simulink model "SWC04_HVPS_DCDCCntrl"  (R2020b)
settings: Solver=FixedStepDiscrete  StartTime=0.0  StopTime=10.0  FixedStep=0.01  RelTol=1e-3
model workspace (MAT data in the model file):
  KSWC07_PDOff_V = Simulink.Parameter
  KSWC07_PDOff_V.Value = 45
  KSWC07_PDOff_V.DataType = 'uint8'
  KSWC07_PDOff_V.Dimensions = [1 1]
  KSWC07_PDOn_V = Simulink.Parameter
  KSWC07_PDOn_V.Value = 15
  KSWC07_PDOn_V.DataType = 'uint8'
  KSWC07_PDOn_V.Dimensions = [1 1]
  NSWC04_B2VSOCEmgncyChgLow_per = Simulink.Parameter
  NSWC04_B2VSOCEmgncyChgLow_per.Value = 30
  NSWC04_B2VSOCEmgncyChgLow_per.DataType = 'uint8'
  NSWC04_B2VSOCEmgncyChgLow_per.Min = 0
  NSWC04_B2VSOCEmgncyChgLow_per.Max = 100
  NSWC04_B2VSOCEmgncyChgLow_per.Dimensions = [1 1]
  NSWC04_KL30EmgncyChgLow_V = Simulink.Parameter
  NSWC04_KL30EmgncyChgLow_V.Value = 95
  NSWC04_KL30EmgncyChgLow_V.DataType = 'uint8'
  NSWC04_KL30EmgncyChgLow_V.Min = 0
  NSWC04_KL30EmgncyChgLow_V.Max = 240
  NSWC04_KL30EmgncyChgLow_V.Dimensions = [1 1]
undefined symbols (not defined in the file): DCDC_14V, HV240V, HV420V, MCUMd_AD, MCUMd_SB, MFbTrq_Off, MRtt_Off, VhSpd_Off, VSUStt_HVOff, VSUStt_HVOn
libraries: simulink x2
settings Model: OrderedModelArguments=off  Creator=Eric  LastModifiedBy=cyw40
settings OptimizationCC: BlockReduction=off  DefaultParameterBehavior=Inlined  UseDivisionForNetSlopeComputation=on  EnhancedBackFolding=on  PassReuseOutputArgsAs=Individual arguments  EfficientFloat2IntCast=on  OptimizeBlockOrder=speed  DifferentSizesBufferReuse=on  OptimizationCustomize=off  EfficientTunableParamExpr=on
settings DebuggingCC: SignalInfNanChecking=error  SignalRangeChecking=error  ReadBeforeWriteMsg=EnableAllAsError  WriteAfterWriteMsg=EnableAllAsError  WriteAfterReadMsg=EnableAllAsError  AlgebraicLoopMsg=error  ArtificialAlgebraicLoopMsg=error  SaveWithDisabledLinksMsg=error  SaveWithParameterizedLinksMsg=error  BlockPriorityViolationMsg=error  SolverPrmCheckMsg=error  InheritedTsInSrcMsg=error  SingleTaskRateTransMsg=error  TasksWithSamePriorityMsg=error  SigSpecEnsureSampleTimeMsg=error  CheckMatrixSingularityMsg=error  IntegerOverflowMsg=error  ParameterUnderflowMsg=error  ParameterPrecisionLossMsg=error  ParameterTunabilityLossMsg=error  UnderSpecifiedDataTypeMsg=error  UnnecessaryDatatypeConvMsg=warning  VectorMatrixConversionMsg=error  SignalLabelMismatchMsg=error  UnconnectedInputMsg=error  UnconnectedOutputMsg=error  UnconnectedLineMsg=error  SFcnCompatibilityMsg=error  UniqueDataStoreMsg=error  BusObjectLabelMismatch=error  RootOutportRequireBusObject=error  AssertControl=DisableAll  ModelReferenceIOMsg=error  ModelReferenceIOMismatchMessage=error  UnknownTsInhSupMsg=error  ModelReferenceDataLoggingMessage=error  StateNameClashWarn=warning  StrictBusMsg=ErrorOnBusTreatedAsVector  NonBusSignalsTreatedAsBus=error  SFInvalidInputDataAccessInChartInitDiag=error  SFTransitionOutsideNaturalParentDiag=error  SFUnreachableExecutionPathDiag=error  SFUndirectedBroadcastEventsDiag=error  SFTransitionActionBeforeConditionDiag=error  SFTemporalDelaySmallerThanSampleTimeDiag=error  SFSelfTransitionDiag=error  SFExecutionAtInitializationDiag=error  SFMachineParentedDataDiag=error  IntegerSaturationMsg=error
settings SFSimCC: CompileTimeRecursionLimit=0  EnableRuntimeRecursion=off  MATLABDynamicMemAlloc=off
settings RTWCC: Description=Embedded Coder  SystemTargetFile=ert.tlc  TemplateMakefile=ert_default_tmf
settings CodeAppCC: ForceParamTrailComments=on  IgnoreCustomStorageClasses=off  OperatorAnnotations=on  SimulinkDataObjDesc=on  SFDataObjDesc=on  MangleLength=4  InsertBlockDesc=on  ReqsInCode=on
settings ERTTargetCC: TargetLangStandard=C99 (ISO)  GenerateSampleERTMain=on  InlinedParameterPlacement=NonHierarchical  ERTCustomFileTemplate=example_file_process.tlc
settings ConfigComp: DVMode=DesignErrorDetection  DVTestSuiteOptimization=Auto  DVDetectDeadLogic=on  DVDetectActiveLogic=on  DVDetectDivisionByZero=off  DVDetectIntegerOverflow=off

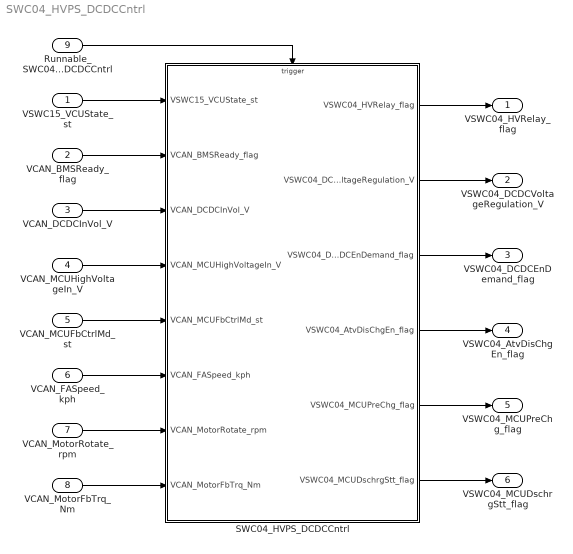
== system SWC04_HVPS_DCDCCntrl ==
  VSWC15_VCUState_st : Inport  OutMin=0  OutMax=13  OutDataTypeStr=uint8  PortDimensions=1
  VCAN_BMSReady_flag : Inport  Port=2  OutMin=0  OutMax=1  OutDataTypeStr=boolean  PortDimensions=1
  VCAN_DCDCInVol_V : Inport  Port=3  OutMin=0  OutMax=500  OutDataTypeStr=uint16  Unit=V  PortDimensions=1
  VCAN_MCUHighVoltageIn_V : Inport  Port=4  OutMin=0  OutMax=500  OutDataTypeStr=uint16  Unit=V  PortDimensions=1
  VCAN_MCUFbCtrlMd_st : Inport  Port=5  OutMin=0  OutMax=4  OutDataTypeStr=uint8  PortDimensions=1
  VCAN_FASpeed_kph : Inport  Port=6  OutMin=0  OutMax=150  OutDataTypeStr=uint8  Unit=km/hr  PortDimensions=1
  VCAN_MotorRotate_rpm : Inport  Port=7  OutMin=0  OutMax=16000  OutDataTypeStr=uint16  Unit=rpm  PortDimensions=1
  VCAN_MotorFbTrq_Nm : Inport  Port=8  OutMin=0  OutMax=225  OutDataTypeStr=uint8  Unit=N*m  PortDimensions=1
  Runnable_SWC04HVPSDCDCCntrl : Inport  Port=9  OutputFunctionCall=on
  SWC04_HVPS_DCDCCntrl : Subsystem
  VSWC04_HVRelay_flag : Outport  OutMin=0  OutMax=1  OutDataTypeStr=boolean  PortDimensions=1
  VSWC04_DCDCVoltageRegulation_V : Outport  Port=2  OutMin=0  OutMax=36  OutDataTypeStr=uint8  Unit=V  PortDimensions=1
  VSWC04_DCDCEnDemand_flag : Outport  Port=3  OutMin=0  OutMax=1  OutDataTypeStr=boolean  PortDimensions=1
  VSWC04_AtvDisChgEn_flag : Outport  Port=4  OutMin=0  OutMax=1  OutDataTypeStr=boolean  PortDimensions=1
  VSWC04_MCUPreChg_flag : Outport  Port=5  OutMin=0  OutMax=1  OutDataTypeStr=boolean  PortDimensions=1
  VSWC04_MCUDschrgStt_flag : Outport  Port=6  OutMin=0  OutMax=1  OutDataTypeStr=boolean  PortDimensions=1
  wires:
  VCAN_BMSReady_flag/1 -> SWC04_HVPS_DCDCCntrl/2(VCAN_BMSReady_flag)
  VCAN_DCDCInVol_V/1 -> SWC04_HVPS_DCDCCntrl/3(VCAN_DCDCInVol_V)
  SWC04_HVPS_DCDCCntrl/2(VSWC04_DCDCVoltageRegulation_V) -> VSWC04_DCDCVoltageRegulation_V/1
  SWC04_HVPS_DCDCCntrl/3(VSWC04_DCDCEnDemand_flag) -> VSWC04_DCDCEnDemand_flag/1
  Runnable_SWC04HVPSDCDCCntrl/1 -> SWC04_HVPS_DCDCCntrl/Trigger
  VSWC15_VCUState_st/1 -> SWC04_HVPS_DCDCCntrl/1(VSWC15_VCUState_st)
  VCAN_MCUHighVoltageIn_V/1 -> SWC04_HVPS_DCDCCntrl/4(VCAN_MCUHighVoltageIn_V)
  SWC04_HVPS_DCDCCntrl/6(VSWC04_MCUDschrgStt_flag) -> VSWC04_MCUDschrgStt_flag/1
  VCAN_MCUFbCtrlMd_st/1 -> SWC04_HVPS_DCDCCntrl/5(VCAN_MCUFbCtrlMd_st)
  SWC04_HVPS_DCDCCntrl/1(VSWC04_HVRelay_flag) -> VSWC04_HVRelay_flag/1
  SWC04_HVPS_DCDCCntrl/5(VSWC04_MCUPreChg_flag) -> VSWC04_MCUPreChg_flag/1
  SWC04_HVPS_DCDCCntrl/4(VSWC04_AtvDisChgEn_flag) -> VSWC04_AtvDisChgEn_flag/1
  VCAN_FASpeed_kph/1 -> SWC04_HVPS_DCDCCntrl/6(VCAN_FASpeed_kph)
  VCAN_MotorRotate_rpm/1 -> SWC04_HVPS_DCDCCntrl/7(VCAN_MotorRotate_rpm)
  VCAN_MotorFbTrq_Nm/1 -> SWC04_HVPS_DCDCCntrl/8(VCAN_MotorFbTrq_Nm)

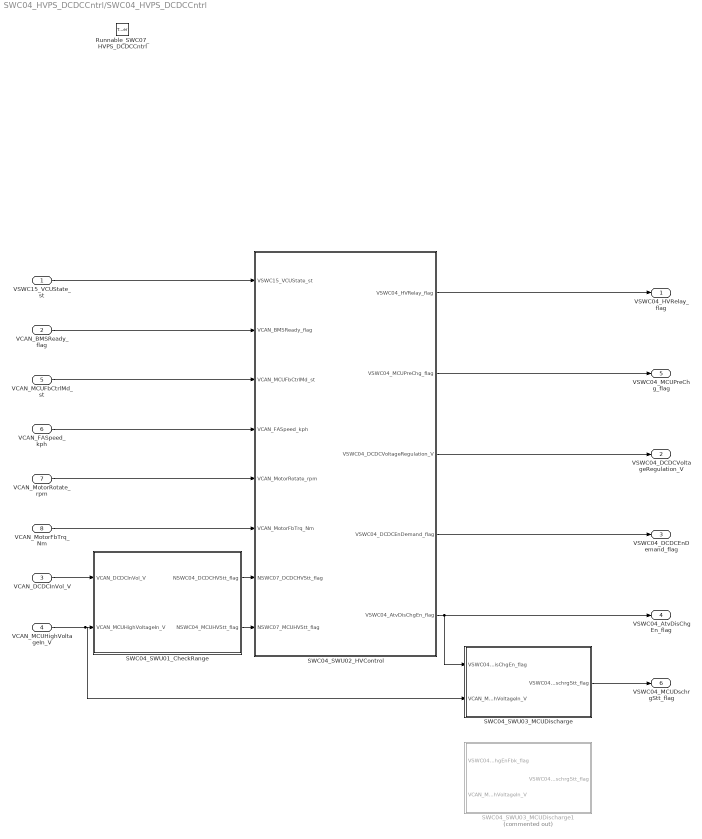
== system SWC04_HVPS_DCDCCntrl/SWC04_HVPS_DCDCCntrl ==
  VSWC15_VCUState_st : Inport
  VCAN_BMSReady_flag : Inport  Port=2
  VCAN_DCDCInVol_V : Inport  Port=3
  VCAN_MCUHighVoltageIn_V : Inport  Port=4
  VCAN_MCUFbCtrlMd_st : Inport  Port=5
  VCAN_FASpeed_kph : Inport  Port=6
  VCAN_MotorRotate_rpm : Inport  Port=7
  VCAN_MotorFbTrq_Nm : Inport  Port=8
  Runnable_SWC07_HVPS_DCDCCntrl : TriggerPort  TriggerType=function-call  VariantControl=Variant
  SWC04_SWU01_CheckRange : Subsystem  TreatAsAtomicUnit=on  RTWFcnName=SWC04_SWU01_CheckRange
      settings: RTWSystemCode=Nonreusable function  RTWFcnNameOpts=User specified
  SWC04_SWU02_HVControl : Subsystem  TreatAsAtomicUnit=on  RTWFcnName=SWC04_SWU02_HVControl
      settings: RTWSystemCode=Nonreusable function  RTWFcnNameOpts=User specified
  SWC04_SWU03_MCUDischarge : Subsystem  TreatAsAtomicUnit=on  RTWFcnName=SWC04_SWU03_MCUDischarge  VariantControl=Choice_1
      settings: RTWSystemCode=Nonreusable function  RTWFcnNameOpts=User specified
  SWC04_SWU03_MCUDischarge1 : Subsystem  Commented=on  VariantControl=Choice_2
  VSWC04_HVRelay_flag : Outport
  VSWC04_DCDCVoltageRegulation_V : Outport  Port=2
  VSWC04_DCDCEnDemand_flag : Outport  Port=3
  VSWC04_AtvDisChgEn_flag : Outport  Port=4
  VSWC04_MCUPreChg_flag : Outport  Port=5
  VSWC04_MCUDschrgStt_flag : Outport  Port=6
  wires:
  SWC04_SWU02_HVControl/3(VSWC04_DCDCVoltageRegulation_V) -> VSWC04_DCDCVoltageRegulation_V/1
  SWC04_SWU02_HVControl/4(VSWC04_DCDCEnDemand_flag) -> VSWC04_DCDCEnDemand_flag/1
  VSWC15_VCUState_st/1 -> SWC04_SWU02_HVControl/1(VSWC15_VCUState_st)
  VCAN_BMSReady_flag/1 -> SWC04_SWU02_HVControl/2(VCAN_BMSReady_flag)
  VCAN_DCDCInVol_V/1 -> SWC04_SWU01_CheckRange/1(VCAN_DCDCInVol_V)
  VCAN_MCUHighVoltageIn_V/1 -> SWC04_SWU03_MCUDischarge/2(VCAN_MCUHighVoltageIn_V), SWC04_SWU01_CheckRange/2(VCAN_MCUHighVoltageIn_V)
  SWC04_SWU02_HVControl/1(VSWC04_HVRelay_flag) -> VSWC04_HVRelay_flag/1
  SWC04_SWU02_HVControl/2(VSWC04_MCUPreChg_flag) -> VSWC04_MCUPreChg_flag/1
  VCAN_MCUFbCtrlMd_st/1 -> SWC04_SWU02_HVControl/3(VCAN_MCUFbCtrlMd_st)
  SWC04_SWU02_HVControl/5(VSWC04_AtvDisChgEn_flag) -> SWC04_SWU03_MCUDischarge/1(VSWC04_AtvDisChgEn_flag), VSWC04_AtvDisChgEn_flag/1
  VCAN_FASpeed_kph/1 -> SWC04_SWU02_HVControl/4(VCAN_FASpeed_kph)
  VCAN_MotorRotate_rpm/1 -> SWC04_SWU02_HVControl/5(VCAN_MotorRotate_rpm)
  VCAN_MotorFbTrq_Nm/1 -> SWC04_SWU02_HVControl/6(VCAN_MotorFbTrq_Nm)
  SWC04_SWU01_CheckRange/1(NSWC04_DCDCHVStt_flag) -> SWC04_SWU02_HVControl/7(NSWC07_DCDCHVStt_flag)
  SWC04_SWU01_CheckRange/2(NSWC04_MCUHVStt_flag) -> SWC04_SWU02_HVControl/8(NSWC07_MCUHVStt_flag)
  SWC04_SWU03_MCUDischarge/1(VSWC04_MCUDschrgStt_flag) -> VSWC04_MCUDschrgStt_flag/1

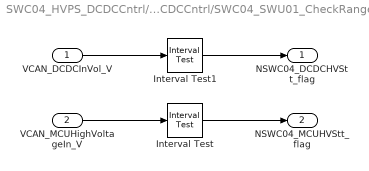
== system SWC04_HVPS_DCDCCntrl/SWC04_HVPS_DCDCCntrl/SWC04_SWU01_CheckRange ==
  VCAN_DCDCInVol_V : Inport
  VCAN_MCUHighVoltageIn_V : Inport  Port=2
  Interval Test : simulink/Logic and Bit Operations/Interval Test  IntervalClosedRight=on  uplimit=HV420V  IntervalClosedLeft=on  lowlimit=HV240V  OutDataTypeStr=boolean
      settings: AttributesFormatString=%<uplimit>~%<lowlimit>
  Interval Test1 : simulink/Logic and Bit Operations/Interval Test  IntervalClosedRight=on  uplimit=HV420V  IntervalClosedLeft=on  lowlimit=HV240V  OutDataTypeStr=boolean
      settings: AttributesFormatString=%<uplimit>~%<lowlimit>
  NSWC04_DCDCHVStt_flag : Outport
  NSWC04_MCUHVStt_flag : Outport  Port=2
  wires:
  Interval Test/1 -> NSWC04_MCUHVStt_flag/1
  Interval Test1/1 -> NSWC04_DCDCHVStt_flag/1
  VCAN_MCUHighVoltageIn_V/1 -> Interval Test/1
  VCAN_DCDCInVol_V/1 -> Interval Test1/1

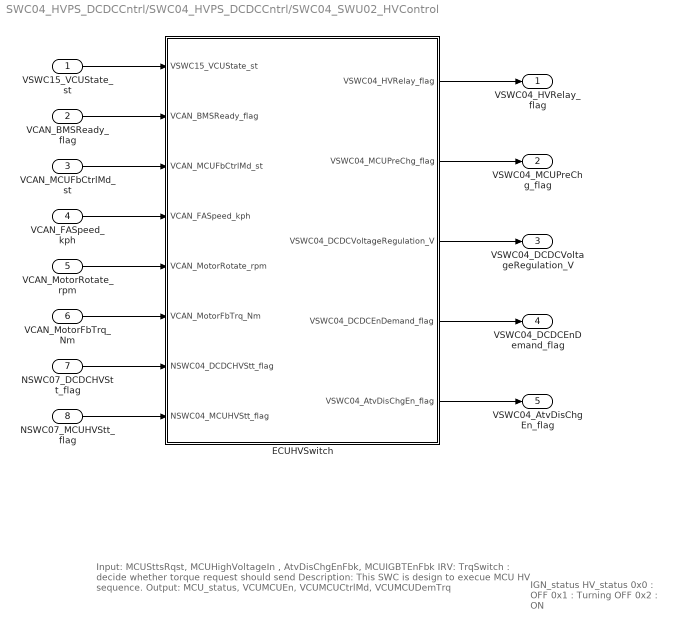
== system SWC04_HVPS_DCDCCntrl/SWC04_HVPS_DCDCCntrl/SWC04_SWU02_HVControl ==
  note: Input:
      | MCUSttsRqst, MCUHighVoltageIn , AtvDisChgEnFbk, MCUIGBTEnFbk
      | IRV:
      | TrqSwitch : decide whether torque request should send
      | Description:
      | This SWC is design to execue MCU HV sequence.
      | Output:
      | MCU_status, VCUMCUEn, VCUMCUCtrlMd, VCUMCUDemTrq
  note: IGN_status
      | HV_status
      | 0x0 : OFF
      | 0x1 : Turning OFF
      | 0x2 : ON
  VSWC15_VCUState_st : Inport
  VCAN_BMSReady_flag : Inport  Port=2
  VCAN_MCUFbCtrlMd_st : Inport  Port=3
  VCAN_FASpeed_kph : Inport  Port=4
  VCAN_MotorRotate_rpm : Inport  Port=5
  VCAN_MotorFbTrq_Nm : Inport  Port=6
  NSWC07_DCDCHVStt_flag : Inport  Port=7
  NSWC07_MCUHVStt_flag : Inport  Port=8
  ECUHVSwitch : Stateflow chart  TreatAsAtomicUnit=on
      settings: PortSchema="{\"entries\":[{\"content\":{\"sides\":[{\"content\":{\"connectorIds\":[\"In1\",\"In2\",\"In8\",\"In4\",\"In5\",\"In6\",\"In3\",\"In7\"]},\"type\":\"ConnectorPlacement.EquallySpacedRectSide\",\"uuid\":\"9266dbf1-70a9-4f04-bd33-da9c8fd394b7\"},{\"content\":{\"connectorIds\":[\"Out4\",\"Out5\",\"Out1\",\"Out2\",\"Out3\"],\"side\":\"RIGHT\"},\"type\":\"ConnectorPlacement.EquallySpacedRectSide\",\"uuid\":\"b1d84704-ffdf-48b3-a93e-c6e208d4a054\"},{\"content\":{\"connectorIds\":[],\"side\":\"TOP\"},\"type\":\"ConnectorPlacement.EquallySpacedRectSide\",\"uuid\":\"22257b4b-f0fe-493f-89ec-3d9780fbdfcd\"}]},\"type\":\"ConnectorPlacement.EquallySpacedConnector\",\"uuid\":\"47fdcc1c-09bf-4f9e-aa31-54a32f75a143\"}],\"packageUris\":[\"http://schema.mathworks.com/mf0/Connector/R2020b\"],\"version\":\"1.0\"}"
  VSWC04_HVRelay_flag : Outport
  VSWC04_MCUPreChg_flag : Outport  Port=2
  VSWC04_DCDCVoltageRegulation_V : Outport  Port=3
  VSWC04_DCDCEnDemand_flag : Outport  Port=4
  VSWC04_AtvDisChgEn_flag : Outport  Port=5
  wires:
  VCAN_BMSReady_flag/1 -> ECUHVSwitch/2(VCAN_BMSReady_flag)
  ECUHVSwitch/1(VSWC04_DCDCVoltageRegulation_V) -> VSWC04_DCDCVoltageRegulation_V/1
  ECUHVSwitch/2(VSWC04_DCDCEnDemand_flag) -> VSWC04_DCDCEnDemand_flag/1
  ECUHVSwitch/4(VSWC04_HVRelay_flag) -> VSWC04_HVRelay_flag/1
  VCAN_MCUFbCtrlMd_st/1 -> ECUHVSwitch/8(VCAN_MCUFbCtrlMd_st)
  ECUHVSwitch/5(VSWC04_MCUPreChg_flag) -> VSWC04_MCUPreChg_flag/1
  ECUHVSwitch/3(VSWC04_AtvDisChgEn_flag) -> VSWC04_AtvDisChgEn_flag/1
  VSWC15_VCUState_st/1 -> ECUHVSwitch/1(VSWC15_VCUState_st)
  VCAN_FASpeed_kph/1 -> ECUHVSwitch/4(VCAN_FASpeed_kph)
  VCAN_MotorRotate_rpm/1 -> ECUHVSwitch/5(VCAN_MotorRotate_rpm)
  VCAN_MotorFbTrq_Nm/1 -> ECUHVSwitch/6(VCAN_MotorFbTrq_Nm)
  NSWC07_DCDCHVStt_flag/1 -> ECUHVSwitch/3(NSWC04_DCDCHVStt_flag)
  NSWC07_MCUHVStt_flag/1 -> ECUHVSwitch/7(NSWC04_MCUHVStt_flag)

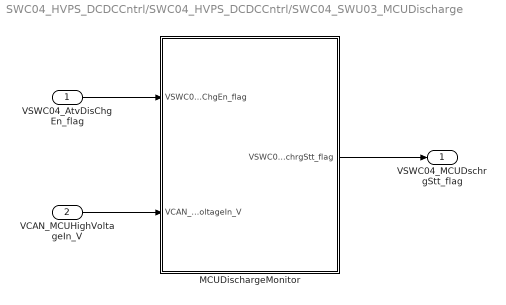
== system SWC04_HVPS_DCDCCntrl/SWC04_HVPS_DCDCCntrl/SWC04_SWU03_MCUDischarge ==
  VSWC04_AtvDisChgEn_flag : Inport
  VCAN_MCUHighVoltageIn_V : Inport  Port=2
  MCUDischargeMonitor : Stateflow chart  TreatAsAtomicUnit=on  VariantControl=Choice
  VSWC04_MCUDschrgStt_flag : Outport
  wires:
  VCAN_MCUHighVoltageIn_V/1 -> MCUDischargeMonitor/2(VCAN_MCUHighVoltageIn_V)
  MCUDischargeMonitor/1(VSWC04_MCUDschrgStt_flag) -> VSWC04_MCUDschrgStt_flag/1
  VSWC04_AtvDisChgEn_flag/1 -> MCUDischargeMonitor/1(VSWC04_AtvDisChgEn_flag)

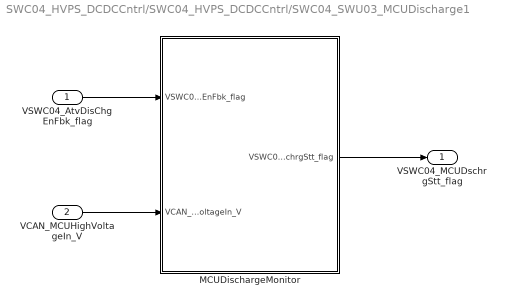
== system SWC04_HVPS_DCDCCntrl/SWC04_HVPS_DCDCCntrl/SWC04_SWU03_MCUDischarge1 ==
  VSWC04_AtvDisChgEnFbk_flag : Inport
  VCAN_MCUHighVoltageIn_V : Inport  Port=2
  MCUDischargeMonitor : Stateflow chart  TreatAsAtomicUnit=on  VariantControl=Choice
  VSWC04_MCUDschrgStt_flag : Outport
  wires:
  VSWC04_AtvDisChgEnFbk_flag/1 -> MCUDischargeMonitor/1(VSWC04_AtvDisChgEnFbk_flag)
  MCUDischargeMonitor/1(VSWC04_MCUDschrgStt_flag) -> VSWC04_MCUDschrgStt_flag/1
  VCAN_MCUHighVoltageIn_V/1 -> MCUDischargeMonitor/2(VCAN_MCUHighVoltageIn_V)

== stateflow chart SWC04_HVPS_DCDCCntrl/SWC04_SWU03_MCUDischarge/MCUDischargeMonitor ==
  state HVOn
  state HVOff
  state Fault
    VSWC04_MCUDschrgStt_flag = false;
  state Finish
    VSWC04_MCUDschrgStt_flag = true;
  (default) -> HVOn
  HVOn -> HVOff : [VSWC04_AtvDisChgEn_flag]
  HVOff -> (junction 50) [order 2] : [after(time+1,tick)]
  HVOff -> (junction 32) [order 1] : [before(time,tick) &&...
      |  VCAN_MCUHighVoltageIn_V < HV50V]
  (junction 50) -> Fault
  (junction 32) -> Finish
  data: VSWC04_AtvDisChgEn_flag input; VCAN_MCUHighVoltageIn_V input; VSWC04_MCUDschrgStt_flag output boolean size=1; HV50V parameter; time constant uint16 size=1 =600

== stateflow chart SWC04_HVPS_DCDCCntrl/SWC04_SWU02_HVControl/ECUHVSwitch ==
  state HVOff
    state Off_start
      Flag1 = false;
    state DCDC_Off
      VSWC04_DCDCEnDemand_flag = false;
    state HV_Off
      VSWC04_HVRelay_flag = false;
    state MCU_Off
      VSWC04_AtvDisChgEn_flag = true;
    state Off_finish
      Flag1 = true;
    (default) -> Off_start
    Off_start -> DCDC_Off : [VCAN_MCUFbCtrlMd_st == MCUMd_AD &&...
        |  VCAN_FASpeed_kph < VhSpd_Off &&...
        |  VCAN_MotorRotate_rpm < MRtt_Off &&...
        |  VCAN_MotorFbTrq_Nm < MFbTrq_Off]
    DCDC_Off -> HV_Off
    HV_Off -> MCU_Off
    MCU_Off -> Off_finish
  state Ready
  state HVOn
    state DCDC_ON [parallel]
      settings: executionOrder=1
      state On_Start
        Flag1 = false;
      state DCDC_On
        VSWC04_DCDCVoltageRegulation_V = DCDC_14V;
        VSWC04_DCDCEnDemand_flag = true;
        Flag1 = true;
      (default) -> HVOn.DCDC_ON.On_Start
      HVOn.DCDC_ON.On_Start -> DCDC_On : [NSWC04_DCDCHVStt_flag]
    state MCU_ON [parallel]
      settings: executionOrder=2
      state On_Start
        Flag2 = false;
      state MCU_On
        VSWC04_MCUPreChg_flag = true;
      state MCU_Fault
        VSWC04_MCUPreChg_flag = false;
      state On_finish
        Flag2 = true;
      (default) -> HVOn.MCU_ON.On_Start
      HVOn.MCU_ON.On_Start -> (junction 210) [order 1] : [before(time,tick) &&...
          |  NSWC04_MCUHVStt_flag]
      HVOn.MCU_ON.On_Start -> (junction 212) [order 2] : [after(time+1,tick)]
      (junction 210) -> MCU_On
      (junction 212) -> MCU_Fault
      MCU_On -> On_finish : [VCAN_MCUFbCtrlMd_st == MCUMd_SB]
  (default) -> Ready
  Ready -> HVOff [order 2] : [VSWC15_VCUState_st == VSUStt_HVOff]
  Ready -> HVOn [order 1] : [VSWC15_VCUState_st == VSUStt_HVOn && ...
      |  VCAN_BMSReady_flag]
      | {
      |  VSWC04_HVRelay_flag = true;
      | }
  HVOn -> Ready : [Flag2 && Flag1]
  HVOff -> Ready : [Flag1]
  data: VSWC15_VCUState_st input; VCAN_BMSReady_flag input; NSWC04_DCDCHVStt_flag input; VCAN_FASpeed_kph input; VCAN_MotorRotate_rpm input; VCAN_MotorFbTrq_Nm input; VSWC04_DCDCVoltageRegulation_V output uint8 size=1; VSWC04_DCDCEnDemand_flag output boolean size=1; DCDC_14V parameter uint8 size=1; NSWC04_MCUHVStt_flag input; VSWC04_AtvDisChgEn_flag output boolean size=1; VSWC04_HVRelay_flag output boolean size=1; VSWC04_MCUPreChg_flag output boolean size=1; Flag1 local boolean size=1; Flag2 local boolean size=1; MCUMd_AD parameter; VCAN_MCUFbCtrlMd_st input; MCUMd_SB parameter; MFbTrq_Off parameter; MRtt_Off parameter; VhSpd_Off parameter; VSUStt_HVOff parameter; VSUStt_HVOn parameter; time constant uint8 size=1 =100

== stateflow chart SWC04_HVPS_DCDCCntrl/SWC04_SWU03_MCUDischarge1/MCUDischargeMonitor ==
  state HVOn
  state Trial
  state HVOff
  state Fault
    VSWC04_MCUDschrgStt_flag = false;
  state Finish
    VSWC04_MCUDschrgStt_flag = true;
  (default) -> HVOn
  HVOn -> HVOff : [VSWC04_AtvDisChgEnFbk_flag]
  Trial -> HVOff
  HVOff -> (junction 50) [order 2] : [after(time+1,tick)]
  HVOff -> (junction 32) [order 1] : [before(time,tick) &&...
      |  VCAN_MCUHighVoltageIn_V < HV50V]
  (junction 50) -> Fault
  (junction 32) -> Finish
  (junction 62) -> Trial
  Fault -> (junction 62) : [after(100,tick)]
  data: VSWC04_AtvDisChgEnFbk_flag input; VCAN_MCUHighVoltageIn_V input; VSWC04_MCUDschrgStt_flag output boolean size=1; HV50V parameter; time constant uint8 size=1 =100
